simulink model "Schemat_ogolny"  (R2021b)
settings: Solver=VariableStepAuto  StartTime=0.0  StopTime=15  RelTol=1e-3
values from neighbouring files (symbols this model uses):
  A_1 = (pi * (1.2 * 15)^2) / 4 / 10000 * size^2    (= 0.101787601976)    [init.m]    (also in init_notebook.m)
  A_2 = (pi * ((1.2 * 15)^2-(1.2*5)^2)) / 4 / 10000 * size^2    (= 0.0904778684234)    [init.m]    (also in init_notebook.m)
  angles = deg2rad (angles)    [init.m]    (also in init_notebook.m)
  F_force = F_aero.*(0.15 + 0.25 * cord + (x/1000).*cos(angles - beta_angles))/0.225    [init.m]    (also in init_notebook.m)
  filter_coef = 100    [init.m]    (also in init_notebook.m)
  m = 8 * 10^(-6) * pi/4 * (5 * 1.2)^2 * 200 * size^3    (= 0.361911473694)    [init.m]    (also in init_notebook.m)
  RAD = deg2rad(A(:,2))    [init.m]    (also in init_notebook.m; rownanie_ruchu.m)
  velocity = transpose(velocity)    [init.m]    (also in init_notebook.m)
  X = A(:,1) / 1000    [init.m]    (also in init_notebook.m; rownanie_ruchu.m = A(:,1))
  x_max = 0.07    [init.m]    (also in init_notebook.m)
  x_min = -0.07    [init.m]    (also in init_notebook.m)
undefined symbols (not defined in the file or in its folder): p_0
libraries: simulink x4, simulink_extras x2, slpidlib x1
settings Model: Creator=01149922  LastModifiedBy=micha
settings SolverCC: AlgebraicLoopSolver=TrustRegion
settings DebuggingCC: SFMachineParentedDataDiag=warning
settings RTWCC: DLArmComputeVersion=20.02.1

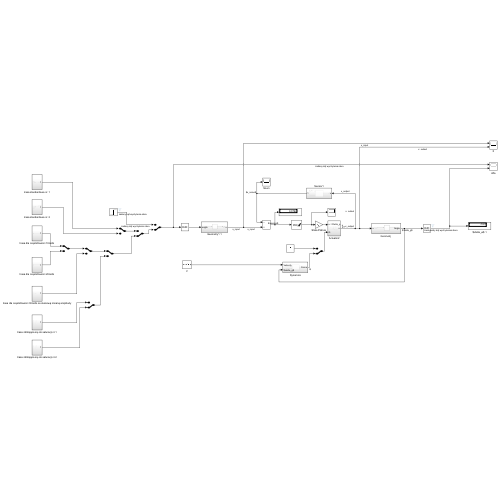
[thumbnail: Simulink's stored preview of the top-level diagram]
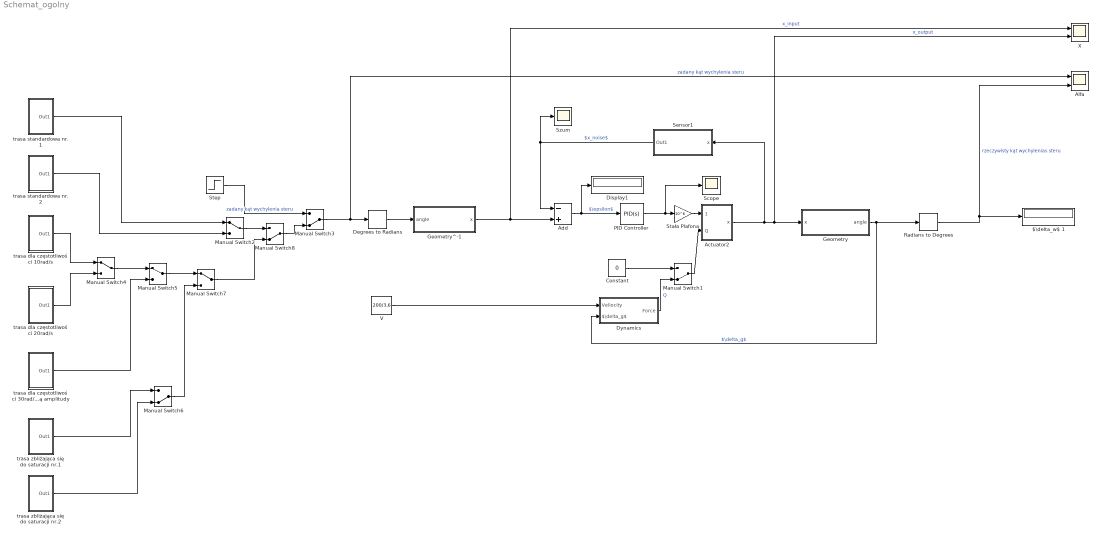
== system Schemat_ogolny ==
  $\delta_w$ 1 : Display
  Actuator2 : Subsystem
  Add : Sum  Inputs=-+
  Alfa : Scope  NumInputPorts=2
  Constant : Constant  Value=0
  Degrees to Radians : simulink_extras/Transformations/Degrees to Radians
  Display1 : Display
  Dynamics : Subsystem
  Geometry : Subsystem
  Geometry^-1 : Subsystem
  Manual Switch{1,3,6,8} (4 alike) : ManualSwitch  CurrentSetting=0
  Manual Switch{2,4..5,7} (4 alike) : ManualSwitch
  PID Controller : slpidlib/PID Controller  Controller=PID  Form=Parallel  TimeDomain=Continuous-time  UseExternalTs=off  SampleTime=-1  IntegratorMethod=Forward Euler  FilterMethod=Forward Euler  ControllerParametersSource=internal  P=-58.2354448652624  I=-33991.1332471453  D=-0.0244992302644784  UseFilter=on  N=1/filter_coef  TunerSelectOption=Frequency Response Based  InitialConditionSource=internal  InitialConditionForIntegrator=0  InitialConditionForFilter=0  DifferentiatorICPrevScaledInput=0  ExternalReset=none  TrackingMode=off  Kt=1  LimitOutput=on  SatLimitsSource=internal  UpperSaturationLimit=x_max  LowerSaturationLimit=x_min  LinearizeAsGain=on  AntiWindupMode=clamping  Kb=1  POutMin=[]  POutMax=[]  IOutMin=[]  IOutMax=[]  DOutMin=[]  DOutMax=[]  NOutMin=[]  NOutMax=[]  SumOutMin=[]  SumOutMax=[]  SaturationOutMin=[]  SaturationOutMax=[]  PParamMin=[]  PParamMax=[]  IParamMin=[]  IParamMax=[]  DParamMin=[]  DParamMax=[]  NParamMin=[]  NParamMax=[]  KbParamMin=[]  KbParamMax=[]  KtParamMin=[]  KtParamMax=[]  KbOutMin=[]  KbOutMax=[]  KtOutMin=[]  KtOutMax=[]  IntegratorOutMin=[]  IntegratorOutMax=[]  FilterOutMin=[]  FilterOutMax=[]  SumI1OutMin=[]  SumI1OutMax=[]  SumI2OutMin=[]  SumI2OutMax=[]  SumI3OutMin=[]  SumI3OutMax=[]  SumI4OutMin=[]  SumI4OutMax=[]  SumDOutMin=[]  SumDOutMax=[]  DifferentiatorOutMin=[]  DifferentiatorOutMax=[]  FilterDiffOutCoefMin=[]  FilterDiffOutCoefMax=[]  ReciprocalOutMin=[]  ReciprocalOutMax=[]  SumDenOutMin=[]  SumDenOutMax=[]  SumNumOutMin=[]  SumNumOutMax=[]  DivideOutMin=[]  DivideOutMax=[]  UdiffTsProdOutMin=[]  UdiffTsProdOutMax=[]  NTsProdOutMin=[]  NTsProdOutMax=[]  UintegralTsProdOutMin=[]  UintegralTsProdOutMax=[]  UngainTsProdOutMin=[]  UngainTsProdOutMax=[]  IntegratorContinuousStateAttributes=''  IntegratorStateMustResolveToSignalObject=off  IntegratorRTWStateStorageClass=Auto  FilterContinuousStateAttributes=''  FilterStateMustResolveToSignalObject=off  FilterRTWStateStorageClass=Auto  ParallelPVariant=InternalParameters  IdealPVariant=Disabled  IVariant=InternalParameters  DVariant=InternalParameters  IntegratorVariant=Continuous  SatVariant=Enabled  AWVariant=ContClampingParallel  PCopyVariant=Disabled  TRVariant=Disabled  FdbkBlocksVariant=Forward  IdealPFdbkVariant=Disabled  SatFdbkVariant=Disabled  DerivativeFilterVariant=ContFilter  NVariant=InternalParameters  NCopyVariant=Disabled  FilterICVariant=InternalICsFilter  IntegratorICVariant=InternalICs  ExternalResetVariant=Disabled  TRSumVariant=Passthrough  SumFdbkVariant=Disabled  SumVariant=Sum_PID  TsampFilterVariant=InternalTs  TsampNgainVariant=Passthrough  TsampIntegralVariant=Passthrough  ExternalSaturationOutDataTypeStr=Inherit: Same as second input
  Radians to Degrees : simulink_extras/Transformations/Radians to Degrees
  Scope : Scope
  Sensor1 : Subsystem
  Stała Plafona : Gain  Gain=10^6
  Step : Step  SampleTime=0
  Szum : Scope
  V : Constant  Value=200/3.6
  X : Scope  NumInputPorts=2
  trasa dla częstotliwości 10rad/s : Subsystem
  trasa dla częstotliwości 20rad/s : Subsystem
  trasa dla częstotliwości 30rad/s ze skokową zmianą amplitudy : Subsystem
  trasa standardowa nr. 1 : Subsystem
  trasa standardowa nr. 2 : Subsystem
  trasa zbliżająca się do saturacji nr.1 : Subsystem
  trasa zbliżająca się do saturacji nr.2 : Subsystem
  wires:
  Add/1 -> Display1/1, PID Controller/1  "$\\epsilon$"
  Actuator2/1(x) -> Sensor1/1(x), X/2, Geometry/1("x ")  "x_output"
  Geometry/1(angle) -> Radians to Degrees/1, Dynamics/2($\delta_g$)  "$\\delta_g$"
  V/1 -> Dynamics/1(Veliocity)
  Degrees to Radians/1 -> Geometry^-1/1(angle)
  Geometry^-1/1(x) -> Add/2, X/1  "x_input"
  Radians to Degrees/1 -> Alfa/2, $\delta_w$ 1/1  "rzeczywisty kąt wychylenias steru"
  PID Controller/1 -> Scope/1, Stała Plafona/1
  Manual Switch3/1 -> Alfa/1, Degrees to Radians/1  "zadany kąt wychylenia steru"
  Dynamics/1(Force) -> Manual Switch1/2  "Q"
  Constant/1 -> Manual Switch1/1
  Manual Switch1/1 -> Actuator2/2(Q)
  Stała Plafona/1 -> Actuator2/1(u = Delta_p)
  Sensor1/1(Out1) -> Szum/1, Add/1  "$x_noise$"
  trasa standardowa nr. 1/1(Out1) -> Manual Switch2/1
  trasa standardowa nr. 2/1(Out1) -> Manual Switch2/2
  Step/1 -> Manual Switch3/1  "zadany kąt wychylenia steru"
  trasa dla częstotliwości 10rad/s/1(Out1) -> Manual Switch4/1
  trasa dla częstotliwości 20rad/s/1(Out1) -> Manual Switch4/2
  trasa zbliżająca się do saturacji nr.1/1(Out1) -> Manual Switch6/1
  trasa zbliżająca się do saturacji nr.2/1(Out1) -> Manual Switch6/2
  Manual Switch4/1 -> Manual Switch5/1
  trasa dla częstotliwości 30rad/s ze skokową zmianą amplitudy/1(Out1) -> Manual Switch5/2
  Manual Switch5/1 -> Manual Switch7/1
  Manual Switch2/1 -> Manual Switch8/1
  Manual Switch8/1 -> Manual Switch3/2
  Manual Switch6/1 -> Manual Switch7/2
  Manual Switch7/1 -> Manual Switch8/2

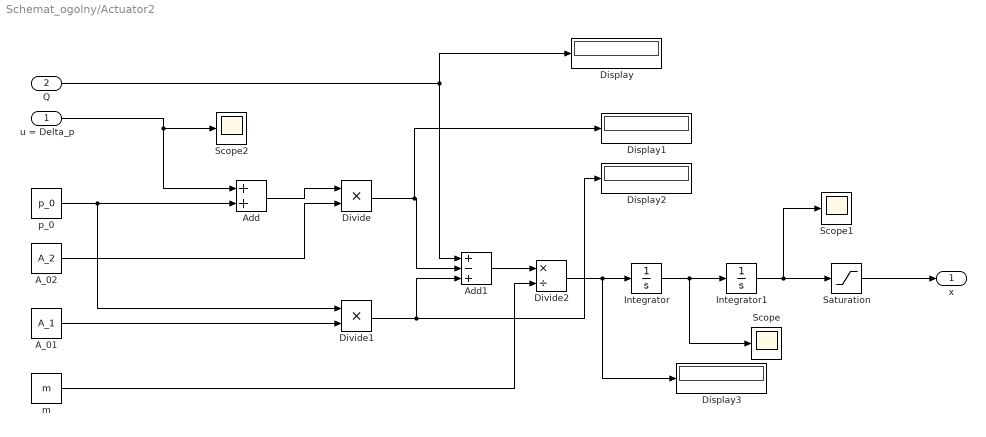
== system Schemat_ogolny/Actuator2 ==
  u = Delta_p : Inport
  Q : Inport  Port=2
  A_01 : Constant  Value=A_1
  A_02 : Constant  Value=A_2
  Add : Sum
  Add1 : Sum  Inputs=+-+
  Display{,1..3} (4 alike) : Display
  Divide : Product  Inputs=**
  Divide1 : Product  Inputs=**
  Divide2 : Product  Inputs=*/
  Integrator : Integrator
  Integrator1 : Integrator
  Saturation : Saturate  UpperLimit=x_max  LowerLimit=x_min
  Scope : Scope
  Scope1 : Scope
  Scope2 : Scope
  m : Constant  Value=m
  p_0 : Constant  Value=p_0
  x : Outport
  wires:
  Add/1 -> Divide/1
  u = Delta_p/1 -> Add/1, Scope2/1
  p_0/1 -> Divide1/1, Add/2
  A_02/1 -> Divide/2
  A_01/1 -> Divide1/2
  Divide/1 -> Display1/1, Add1/2
  Divide1/1 -> Display2/1, Add1/3
  Q/1 -> Add1/1, Display/1
  Add1/1 -> Divide2/1
  m/1 -> Divide2/2
  Divide2/1 -> Display3/1, Integrator/1
  Integrator/1 -> Scope/1, Integrator1/1
  Integrator1/1 -> Scope1/1, Saturation/1
  Saturation/1 -> x/1

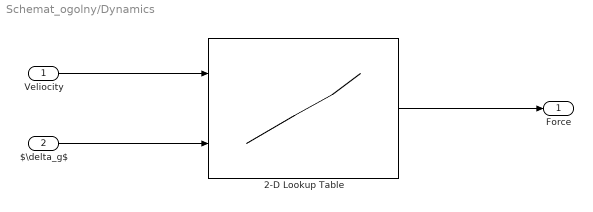
== system Schemat_ogolny/Dynamics ==
  Veliocity : Inport
  $\delta_g$ : Inport  Port=2
  2-D Lookup Table : Lookup_n-D  BreakpointsForDimension1=velocity  BreakpointsForDimension2=angles  Table=F_force  InternalRulePriority=Speed  RndMeth=Simplest  InputSameDT=on
      settings: InputPortMap=u0,u1
  Force : Outport
  wires:
  $\delta_g$/1 -> 2-D Lookup Table/2
  Veliocity/1 -> 2-D Lookup Table/1
  2-D Lookup Table/1 -> Force/1

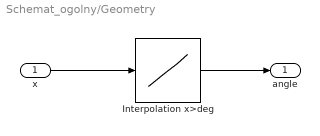
== system Schemat_ogolny/Geometry ==
  "x " : Inport
  Interpolation x>deg : Lookup_n-D  NumberOfTableDimensions=1  BreakpointsForDimension1=X  Table=RAD  InternalRulePriority=Speed  RndMeth=Simplest  InputSameDT=on
  angle : Outport
  wires:
  "x "/1 -> Interpolation x>deg/1
  Interpolation x>deg/1 -> angle/1

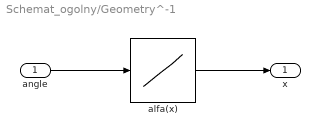
== system Schemat_ogolny/Geometry^-1 ==
  angle : Inport
  alfa(x) : Lookup_n-D  NumberOfTableDimensions=1  BreakpointsForDimension1=RAD  Table=X  InternalRulePriority=Speed  RndMeth=Simplest  InputSameDT=on
  x : Outport
  wires:
  angle/1 -> alfa(x)/1
  alfa(x)/1 -> x/1

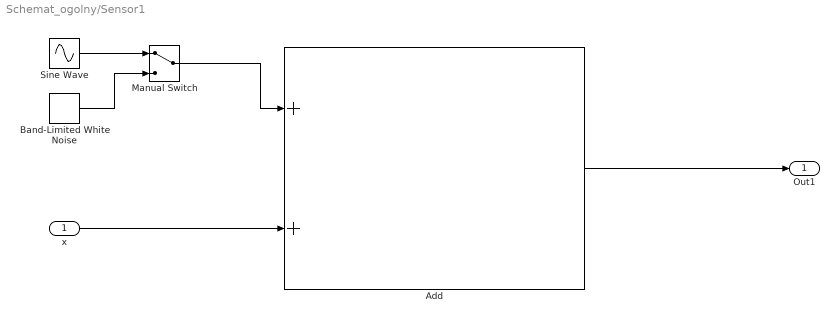
== system Schemat_ogolny/Sensor1 ==
  x : Inport
  Add : Sum
  Band-Limited White Noise : simulink/Sources/Band-Limited White Noise  Cov=filter_coef  Ts=0.0001  seed=[23341]
  Manual Switch : ManualSwitch
  Sine Wave : Sin  Amplitude=filter_coef  Frequency=10^(-4)  SampleTime=0
  Out1 : Outport
  wires:
  Add/1 -> Out1/1
  x/1 -> Add/2
  Manual Switch/1 -> Add/1
  Band-Limited White Noise/1 -> Manual Switch/2
  Sine Wave/1 -> Manual Switch/1

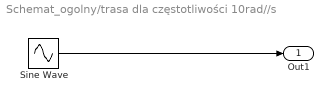
== system Schemat_ogolny/trasa dla częstotliwości 10rad//s ==
  Sine Wave : Sin  Amplitude=14  Frequency=10  SampleTime=0
  Out1 : Outport
  wires:
  Sine Wave/1 -> Out1/1

== system Schemat_ogolny/trasa dla częstotliwości 20rad//s ==
  Sine Wave : Sin  Amplitude=14  Frequency=20  SampleTime=0
  Out1 : Outport
  wires:
  Sine Wave/1 -> Out1/1

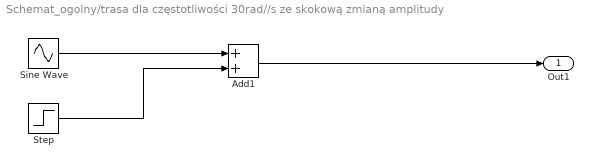
== system Schemat_ogolny/trasa dla częstotliwości 30rad//s ze skokową zmianą amplitudy ==
  Add1 : Sum
  Sine Wave : Sin  Amplitude=8  Frequency=30  SampleTime=0
  Step : Step  Time=2  After=5  SampleTime=0
  Out1 : Outport
  wires:
  Add1/1 -> Out1/1
  Sine Wave/1 -> Add1/1
  Step/1 -> Add1/2

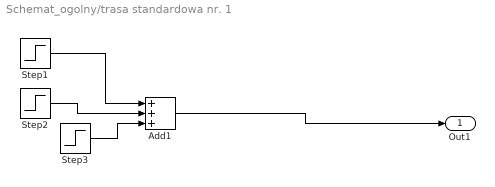
== system Schemat_ogolny/trasa standardowa nr. 1 ==
  Add1 : Sum  Inputs=+++
  Step1 : Step  Time=0.5  Before=2  After=-2  SampleTime=0
  Step2 : Step  After=3  SampleTime=0
  Step3 : Step  Time=2  After=6  SampleTime=0
  Out1 : Outport
  wires:
  Step1/1 -> Add1/1
  Step2/1 -> Add1/2
  Add1/1 -> Out1/1
  Step3/1 -> Add1/3

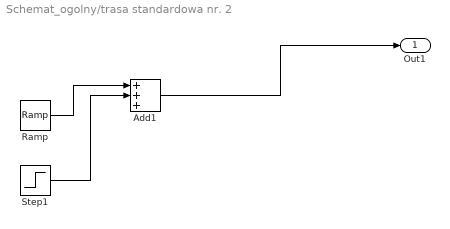
== system Schemat_ogolny/trasa standardowa nr. 2 ==
  Add1 : Sum  Inputs=+++
  Ramp : simulink/Sources/Ramp  slope=2  start=0  InitialOutput=-3
  Step1 : Step  Time=0.5  After=4  SampleTime=0
  Out1 : Outport
  wires:
  Add1/1 -> Out1/1
  Step1/1 -> Add1/2
  Ramp/1 -> Add1/1

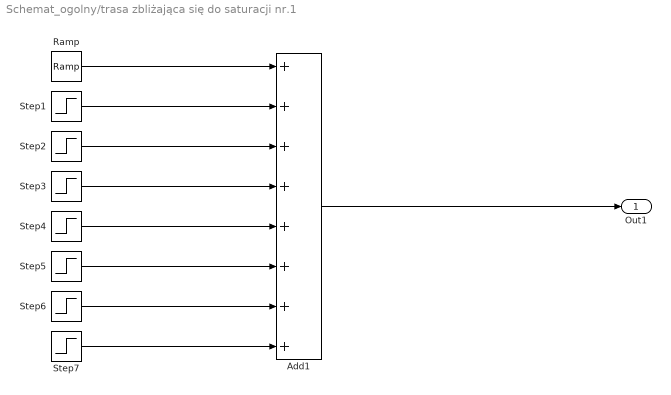
== system Schemat_ogolny/trasa zbliżająca się do saturacji nr.1 ==
  Add1 : Sum  Inputs=++++++++
  Ramp : simulink/Sources/Ramp  slope=1  start=0  InitialOutput=0
  Step1 : Step  Time=2  After=-2  SampleTime=0
  Step2 : Step  Time=4  SampleTime=0
  Step3 : Step  Time=7  After=3  SampleTime=0
  Step4 : Step  Time=8  After=-.5  SampleTime=0
  Step5 : Step  Time=10  After=-3  SampleTime=0
  Step6 : Step  Time=12  After=-0.25  SampleTime=0
  Step7 : Step  Time=14  After=3  SampleTime=0
  Out1 : Outport
  wires:
  Add1/1 -> Out1/1
  Step1/1 -> Add1/2
  Ramp/1 -> Add1/1
  Step2/1 -> Add1/3
  Step3/1 -> Add1/4
  Step4/1 -> Add1/5
  Step6/1 -> Add1/7
  Step5/1 -> Add1/6
  Step7/1 -> Add1/8

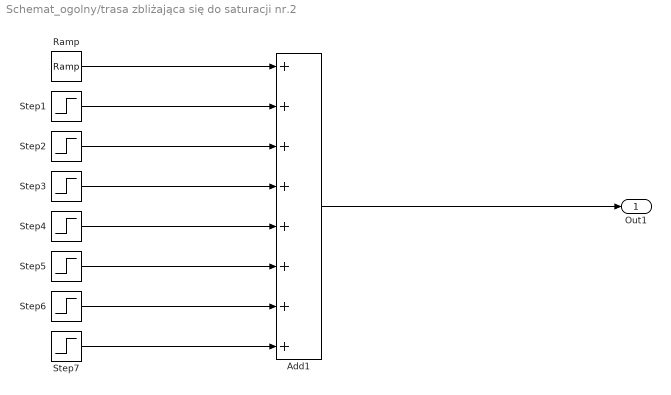
== system Schemat_ogolny/trasa zbliżająca się do saturacji nr.2 ==
  Add1 : Sum  Inputs=++++++++
  Ramp : simulink/Sources/Ramp  slope=1  start=0  InitialOutput=0
  Step1 : Step  Time=2  After=-7  SampleTime=0
  Step2 : Step  Time=4  After=5  SampleTime=0
  Step3 : Step  Time=7  After=10  SampleTime=0
  Step4 : Step  Time=8  After=-2  SampleTime=0
  Step5 : Step  Time=10  After=-10  SampleTime=0
  Step6 : Step  Time=12  After=-0.5  SampleTime=0
  Step7 : Step  Time=14  After=10  SampleTime=0
  Out1 : Outport
  wires:
  Step6/1 -> Add1/7
  Step1/1 -> Add1/2
  Ramp/1 -> Add1/1
  Add1/1 -> Out1/1
  Step7/1 -> Add1/8
  Step2/1 -> Add1/3
  Step4/1 -> Add1/5
  Step3/1 -> Add1/4
  Step5/1 -> Add1/6
